simulink library "lib_dGrid"  (R2023b)
settings: Solver=VariableStepAuto  StartTime=0.0  StopTime=10.0  RelTol=1e-3
values from neighbouring files (symbols this model uses):
  C_PM = 10e-3    (= 0.01)    [my_MMC_param.m]
  Cbase = 1/Zbase/wb    (= 3.10849498226e-05)    [my_MMC_param.m]
  f0 = 50/fb    (= 1)    [my_MMC_param.m]
  Fn_filter = 1000    [my_MMC_param.m]
  Fnom = 50    [my_MMC_param.m]
  GFL_APC = 1    [Analysis_Main.m]    (also in initSimu.m; my_MMC_param.m)
  GFL_DVC = 2    [Analysis_Main.m]    (also in initSimu.m; my_MMC_param.m)
  GFM_APC = 3; (values programmed in EMT models)    [Analysis_Main.m]    (also in initSimu.m; my_MMC_param.m = 3)
  GFM_VF = 0    [my_MMC_param.m]
  Ibase = 2*Sbase/(3*Ubase)    [my_MMC_param.m]
  Idcb = Sbase/Udcb    [my_MMC_param.m]
  Ki_Iccsc = 5.15    [my_MMC_param.m]
  Ki_Ireg = CCCTRL.CC.ki    [my_MMC_param.m]
  Ki_Izscc = 100    [my_MMC_param.m]
  Ki_PLL = 1/(CCCTRL.PLL.v0*CCCTRL.PLL.T^2)    [my_MMC_param.m]
  Ki_Preg = 1.0*10    (= 10)    [my_MMC_param.m]
  Ki_Qreg = 1.0*10    (= 10)    [my_MMC_param.m]
  Ki_VAC_GFL = 50    [my_MMC_param.m]
  Ki_VACreg = 10    [my_MMC_param.m]
  Ki_VDCreg = 10    [my_MMC_param.m]
  Ki_WtReg = Kp_WtReg / 0.025    (= 1600)    [my_MMC_param.m]
  Kp_Iccsc = 0.21    [my_MMC_param.m]
  Kp_Ireg = CCCTRL.CC.kp    [my_MMC_param.m]
  Kp_Izscc = 10    [my_MMC_param.m]
  Kp_PLL = 2/CCCTRL.PLL.v0/CCCTRL.PLL.T    [my_MMC_param.m]
  Kp_Preg = 0.5/3*1    (= 0.166666666667)    [my_MMC_param.m]
  Kp_Qreg = 0.5/3*1    (= 0.166666666667)    [my_MMC_param.m]
  Kp_VAC_GFL = 0.5    [my_MMC_param.m]
  Kp_VACreg = 0.01    [my_MMC_param.m]
  Kp_VDCreg = 1    [my_MMC_param.m]
  Kp_WtReg = 40    [my_MMC_param.m]
  Kpv_GFM = 1    [my_MMC_param.m]
  Kpwm = 0.5    [my_MMC_param.m]
  Larm = Larm_pu*(Zbase/wb)    (= 0.0488923985178)    [my_MMC_param.m]
  Lff = Larm_pu/2    (= 0.075)    [my_MMC_param.m]
  Limits_Ireg = [ 2.0  -2.0]    [my_MMC_param.m]
  Limits_Preg = [ 2, -2 ]    [my_MMC_param.m]
  Limits_Qreg = 2*[ 0.42, -0.42 ]    [my_MMC_param.m]
  Limits_VACreg = [ 1.3  -1.3]    [my_MMC_param.m]
  Limits_VDCreg = [ 2.0  -2.0]    [my_MMC_param.m]
  MMC1 = MMC    [Analysis_Main.m]    (also in initSimu.m)
  Nb_PM = 400    [my_MMC_param.m]
  PhaseDelay = 1.0*Ts_Control*2*pi*50    (= 0.0628318530718)    [my_MMC_param.m]
  Pnom = 1000e6    (= 1000000000)    [my_MMC_param.m]
  Rarm = Rarm_pu*Zbase    (= 0.1536)    [my_MMC_param.m]
  Slope_Pref = 0.5    [my_MMC_param.m]
  Slope_Qref = 0.5    [my_MMC_param.m]
  Slope_Vdc_ref = Vnom_dc/2    (= 320000)    [my_MMC_param.m]
  Tdeblock = 1.5    [my_MMC_param.m]
  Ton_CROSSreg = Ton_PQreg+3    (= 7)    [my_MMC_param.m]
  Ton_PQreg = 4    [my_MMC_param.m]
  Ton_VDCreg = 1.5    [my_MMC_param.m]
  Ts = Ts_Control    (= 0.0002)    [my_MMC_param.m]
  Ts_Control = Ts_Power*2    (= 0.0002)    [my_MMC_param.m]
  Ts_Power = 20e-6 * 5    (= 0.0001)    [my_MMC_param.m]
  Ubase = sqrt(2/3)*Vnom_sec    [my_MMC_param.m]
  Udcb = 2*Ubase    [my_MMC_param.m]
  Vc0_PM = 0    [my_MMC_param.m]
  Vnom_dc = 640e3    (= 640000)    [my_MMC_param.m]
  Vnom_sec = 320e3    (= 320000)    [my_MMC_param.m]
  wb = 2*pi*fb    (= 314.159265359)    [my_MMC_param.m]
  Wt_ref_pu = 0.5 * C_PM * (Vnom_dc/Nb_PM)^2 * Nb_PM * 6 / Pnom    (= 0.03072)    [my_MMC_param.m]
undefined symbols (not defined in the file or in its folder): ControlSampleTime, DiscIntNeverNeededParam, MMC, PLL, VSM
libraries: simulink x50, spsCurrentMeasurementLib x20, spsSecondOrderFilterLib x20, spsDiodeLib x12, spsControlledVoltageSourceLib x12, spsSeriesRLCBranchLib x10, spsFirstOrderFilterLib x9, spsVoltageMeasurementLib x8, spsMeanLib x7, FriedrichLibrary x6, $bdroot x6, powerlib_extras x4
(part 8 of 8)

== system lib_dGrid/MMC-configurable control modes/MMC Control/PLL, Measurements and Transformation/from DDSRF-PLL/PT1 as IIR1 ==
  U : Inport
  Gain : Gain  Gain=K*T/(T+2*tau)  SampleTime=T
  Gain1 : Gain  Gain=K*T/(T+2*tau)
  Gain2 : Gain  Gain=(T-2*tau)/(T+2*tau)
  Sum : Sum  Inputs=|++
  Sum1 : Sum  Inputs=+|-
  Unit Delay : UnitDelay  InitialCondition=Init  SampleTime=T  HasFrameUpgradeWarning=on
  Unit Delay1 : UnitDelay  InitialCondition=Init*K  SampleTime=T  HasFrameUpgradeWarning=on
  Y : Outport  VectorParamsAs1DForOutWhenUnconnected=off
  wires:
  Gain2/1 -> Sum1/2
  Sum1/1 -> Sum/2
  Gain1/1 -> Sum1/1
  Unit Delay1/1 -> Gain2/1
  Sum/1 -> Y/1, Unit Delay1/1
  Gain/1 -> Sum/1
  Unit Delay/1 -> Gain1/1
  U/1 -> Gain/1, Unit Delay/1

== system lib_dGrid/MMC-configurable control modes/MMC Control/PLL, Measurements and Transformation/from DDSRF-PLL/ab0->dq0 SinCos ==
  ab0 : Inport
  sincos : Inport  Port=2
  Demux : Demux  Outputs=3
  Demux1 : Demux  Outputs=2
  Mux : Mux  Inputs=3
  Product{,1..3} (4 alike) : Product
  Subtract : Sum
  Subtract1 : Sum  Inputs=-+
  dq0 : Outport  VectorParamsAs1DForOutWhenUnconnected=off
  wires:
  Mux/1 -> dq0/1
  Demux/3 -> Mux/3
  Demux/1 -> Product2/2, Product/2
  ab0/1 -> Demux/1
  sincos/1 -> Demux1/1
  Demux/2 -> Product1/2, Product3/2
  Demux1/2 -> Product3/1, Product/1
  Demux1/1 -> Product2/1, Product1/1
  Product/1 -> Subtract/1
  Product1/1 -> Subtract/2
  Product2/1 -> Subtract1/1
  Product3/1 -> Subtract1/2
  Subtract1/1 -> Mux/2
  Subtract/1 -> Mux/1

== system lib_dGrid/MMC-configurable control modes/MMC Control/PLL, Measurements and Transformation/from DDSRF-PLL/ab0->dq0 SinCos  ==
  ab0 : Inport
  sincos : Inport  Port=2
  Demux : Demux  Outputs=3
  Demux1 : Demux  Outputs=2
  Mux : Mux  Inputs=3
  Product{,1..3} (4 alike) : Product
  Subtract : Sum
  Subtract1 : Sum  Inputs=-+
  dq0 : Outport  VectorParamsAs1DForOutWhenUnconnected=off
  wires:
  Mux/1 -> dq0/1
  Demux/3 -> Mux/3
  Demux/1 -> Product2/2, Product/2
  ab0/1 -> Demux/1
  sincos/1 -> Demux1/1
  Demux/2 -> Product1/2, Product3/2
  Demux1/2 -> Product3/1, Product/1
  Demux1/1 -> Product2/1, Product1/1
  Product/1 -> Subtract/1
  Product1/1 -> Subtract/2
  Product2/1 -> Subtract1/1
  Product3/1 -> Subtract1/2
  Subtract1/1 -> Mux/2
  Subtract/1 -> Mux/1

== system lib_dGrid/MMC-configurable control modes/MMC Control/PLL, Measurements and Transformation/from DDSRF-PLL/dq0->ab0 SinCos ==
  ab0 : Inport
  sincos : Inport  Port=2
  Demux : Demux  Outputs=3
  Demux1 : Demux  Outputs=2
  Mux : Mux  Inputs=3
  Product{,1..3} (4 alike) : Product
  Subtract : Sum  Inputs=+-
  Subtract1 : Sum
  dq0 : Outport  VectorParamsAs1DForOutWhenUnconnected=off
  wires:
  Subtract/1 -> Mux/1
  Subtract1/1 -> Mux/2
  Product3/1 -> Subtract1/2
  Product2/1 -> Subtract1/1
  Product1/1 -> Subtract/2
  Product/1 -> Subtract/1
  Demux1/1 -> Product1/1, Product2/1
  Demux1/2 -> Product/1, Product3/1
  Demux/2 -> Product3/2, Product1/2
  sincos/1 -> Demux1/1
  ab0/1 -> Demux/1
  Demux/1 -> Product/2, Product2/2
  Demux/3 -> Mux/3
  Mux/1 -> dq0/1

== system lib_dGrid/MMC-configurable control modes/MMC Control/PLL, Measurements and Transformation/from DDSRF-PLL/dq0->ab0 SinCos  ==
  ab0 : Inport
  sincos : Inport  Port=2
  Demux : Demux  Outputs=3
  Demux1 : Demux  Outputs=2
  Mux : Mux  Inputs=3
  Product{,1..3} (4 alike) : Product
  Subtract : Sum  Inputs=+-
  Subtract1 : Sum
  dq0 : Outport  VectorParamsAs1DForOutWhenUnconnected=off
  wires:
  Subtract/1 -> Mux/1
  Subtract1/1 -> Mux/2
  Product3/1 -> Subtract1/2
  Product2/1 -> Subtract1/1
  Product1/1 -> Subtract/2
  Product/1 -> Subtract/1
  Demux1/1 -> Product1/1, Product2/1
  Demux1/2 -> Product/1, Product3/1
  Demux/2 -> Product3/2, Product1/2
  sincos/1 -> Demux1/1
  ab0/1 -> Demux/1
  Demux/1 -> Product/2, Product2/2
  Demux/3 -> Mux/3
  Mux/1 -> dq0/1

== system lib_dGrid/MMC-configurable control modes/MMC Control/VSM Control/Inner Loop Control/CC ==
  Error : Inport  SampleTime=Ts
  Discrete-Time Integrator : DiscreteIntegrator  InitialCondition=Init  SampleTime=Ts  LimitOutput=on  UpperSaturationLimit=UpperLimit  LowerSaturationLimit=LowerLimit  ICPrevOutput=DiscIntNeverNeededParam  ICPrevScaledInput=DiscIntNeverNeededParam
  Kp4 : Gain  Gain=Kp  SaturateOnIntegerOverflow=on  SampleTime=Ts  OutDataTypeStr=Inherit: Same as input  ParamDataTypeStr=Inherit: Same as input
  Kp5 : Gain  Gain=Ki  SaturateOnIntegerOverflow=on  SampleTime=Ts  OutDataTypeStr=Inherit: Same as input  ParamDataTypeStr=Inherit: Same as input
  Saturation2 : Saturate  UpperLimit=UpperLimit  LowerLimit=LowerLimit  SampleTime=Ts
  Sum6 : Sum  InputSameDT=on  SaturateOnIntegerOverflow=on  SampleTime=Ts  OutDataTypeStr=Inherit: Same as first input
  Zero-Order Hold : ZeroOrderHold  SampleTime=Ts
  Out : Outport  SampleTime=Ts  InitialOutput=0  VectorParamsAs1DForOutWhenUnconnected=off
  wires:
  Zero-Order Hold/1 -> Sum6/1
  Error/1 -> Kp5/1, Kp4/1
  Sum6/1 -> Saturation2/1
  Kp4/1 -> Zero-Order Hold/1
  Discrete-Time Integrator/1 -> Sum6/2
  Saturation2/1 -> Out/1
  Kp5/1 -> Discrete-Time Integrator/1

== system lib_dGrid/MMC-configurable control modes/MMC Control/VSM Control/Inner Loop Control/CC  ==
  Error : Inport  SampleTime=Ts
  Discrete-Time Integrator : DiscreteIntegrator  InitialCondition=Init  SampleTime=Ts  LimitOutput=on  UpperSaturationLimit=UpperLimit  LowerSaturationLimit=LowerLimit  ICPrevOutput=DiscIntNeverNeededParam  ICPrevScaledInput=DiscIntNeverNeededParam
  Kp4 : Gain  Gain=Kp  SaturateOnIntegerOverflow=on  SampleTime=Ts  OutDataTypeStr=Inherit: Same as input  ParamDataTypeStr=Inherit: Same as input
  Kp5 : Gain  Gain=Ki  SaturateOnIntegerOverflow=on  SampleTime=Ts  OutDataTypeStr=Inherit: Same as input  ParamDataTypeStr=Inherit: Same as input
  Saturation2 : Saturate  UpperLimit=UpperLimit  LowerLimit=LowerLimit  SampleTime=Ts
  Sum6 : Sum  InputSameDT=on  SaturateOnIntegerOverflow=on  SampleTime=Ts  OutDataTypeStr=Inherit: Same as first input
  Zero-Order Hold : ZeroOrderHold  SampleTime=Ts
  Out : Outport  SampleTime=Ts  InitialOutput=0  VectorParamsAs1DForOutWhenUnconnected=off
  wires:
  Zero-Order Hold/1 -> Sum6/1
  Error/1 -> Kp5/1, Kp4/1
  Sum6/1 -> Saturation2/1
  Kp4/1 -> Zero-Order Hold/1
  Discrete-Time Integrator/1 -> Sum6/2
  Saturation2/1 -> Out/1
  Kp5/1 -> Discrete-Time Integrator/1

== system lib_dGrid/MMC-configurable control modes/MMC Control/VSM Control/VSM1/Angle Integrator [SI] ==
  omega : Inport
  phi0 : Inport  Port=2
  Bias : Bias  Bias=-2*pi  SaturateOnIntegerOverflow=off
  Bias1 : Bias  Bias=2*pi  SaturateOnIntegerOverflow=off
  Delay : Delay  DelayLength=1  InitialConditionSource=Input port  SampleTime=Ts
      settings: InputPortMap=u0,p4
  Gain3 : Gain  Gain=Ts
  Sum : Sum  Inputs=|++
  Switch : Switch  Criteria=u2 > Threshold  Threshold=pi  SaturateOnIntegerOverflow=off  InputSameDT=off
  Switch1 : Switch  Threshold=-pi  SaturateOnIntegerOverflow=off  InputSameDT=off
  phi : Outport  VectorParamsAs1DForOutWhenUnconnected=off
  wires:
  Switch1/1 -> Delay/1
  Bias1/1 -> Switch1/3
  Switch/1 -> Switch1/2, Bias1/1, Switch1/1
  Delay/1 -> phi/1, Sum/2
  Sum/1 -> Bias/1, Switch/2, Switch/3
  Bias/1 -> Switch/1
  Gain3/1 -> Sum/1
  omega/1 -> Gain3/1
  phi0/1 -> Delay/2

== system lib_dGrid/MMC-configurable control modes/MMC Control/VSM Control/Virtual circuit daniel style1/transient rv (HP)1 -dd's form ==
  In1 : Inport
  Add : Sum  Inputs=+-
  Constant : Constant  Value=tau
  Delay2 : Delay  DelayLength=1  SampleTime=TS
  Divide : Product  Inputs=*/
  Gain : Gain  Gain=TS
  Gain1 : Gain
  Sum : Sum  Inputs=|++
  Sum2 : Sum  Inputs=|+-
  Out1 : Outport  VectorParamsAs1DForOutWhenUnconnected=off
  wires:
  Delay2/1 -> Add/2, Sum/2, Sum2/2
  Gain1/1 -> Add/1
  Sum/1 -> Delay2/1
  In1/1 -> Sum2/1, Gain1/1
  Add/1 -> Out1/1
  Divide/1 -> Sum/1
  Constant/1 -> Divide/2
  Sum2/1 -> Gain/1
  Gain/1 -> Divide/1

== system lib_dGrid/MMC-configurable control modes/MMC Control/VSM Control/Virtual circuit daniel style1/transient rv (HP)1 yz's form ==
  In1 : Inport
  Add : Sum  Inputs=+-
  Gain1 : Gain
  Low-Pass Filter (Discrete or Continuous) : eeGeneralControl/Low-Pass Filter (Discrete or Continuous)  K=1  T=tau  B=inf  A=-inf  init_option=Inherited from block input  x0=0  Ts=TS
  Out1 : Outport  VectorParamsAs1DForOutWhenUnconnected=off
  wires:
  Gain1/1 -> Add/1
  In1/1 -> Low-Pass Filter (Discrete or Continuous)/1, Gain1/1
  Add/1 -> Out1/1
  Low-Pass Filter (Discrete or Continuous)/1 -> Add/2

== system lib_dGrid/MMC-configurable control modes/MMC Control/VSM Control/Virtual circuit daniel style1/transient rv (HP)2 (dd's form) ==
  In1 : Inport
  Add : Sum  Inputs=+-
  Constant : Constant  Value=tau
  Delay2 : Delay  DelayLength=1  SampleTime=TS
  Divide : Product  Inputs=*/
  Gain : Gain  Gain=TS
  Gain1 : Gain
  Sum : Sum  Inputs=|++
  Sum2 : Sum  Inputs=|+-
  Out1 : Outport  VectorParamsAs1DForOutWhenUnconnected=off
  wires:
  Gain/1 -> Divide/1
  Sum2/1 -> Gain/1
  Constant/1 -> Divide/2
  Divide/1 -> Sum/1
  Add/1 -> Out1/1
  In1/1 -> Gain1/1, Sum2/1
  Sum/1 -> Delay2/1
  Gain1/1 -> Add/1
  Delay2/1 -> Sum2/2, Sum/2, Add/2

== system lib_dGrid/TL-VSC-configurable control modes/VSC Control/PLL, Measurements and Transformation/Symmetrical PLL/Angle Integrator [SI] ==
  omega : Inport
  phi0 : Inport  Port=2
  Bias : Bias  Bias=-2*pi  SaturateOnIntegerOverflow=off
  Bias1 : Bias  Bias=2*pi  SaturateOnIntegerOverflow=off
  Delay : Delay  DelayLength=1  InitialConditionSource=Input port  SampleTime=Ts
      settings: InputPortMap=u0,p4
  Gain3 : Gain  Gain=Ts
  Sum : Sum  Inputs=|++
  Switch : Switch  Criteria=u2 > Threshold  Threshold=pi  SaturateOnIntegerOverflow=off  InputSameDT=off
  Switch1 : Switch  Threshold=-pi  SaturateOnIntegerOverflow=off  InputSameDT=off
  phi : Outport  VectorParamsAs1DForOutWhenUnconnected=off
  wires:
  Switch1/1 -> Delay/1
  Bias1/1 -> Switch1/3
  Switch/1 -> Switch1/2, Bias1/1, Switch1/1
  Delay/1 -> phi/1, Sum/2
  Sum/1 -> Bias/1, Switch/2, Switch/3
  Bias/1 -> Switch/1
  Gain3/1 -> Sum/1
  omega/1 -> Gain3/1
  phi0/1 -> Delay/2

== system lib_dGrid/TL-VSC-configurable control modes/VSC Control/PLL, Measurements and Transformation/Symmetrical PLL/PhN->ab0 ==
  PhN : Inport
  AlphaBetaNull Transformation : Gain  Gain="[2/3   -1/3    -1/3;   0   1/sqrt(3) -1/sqrt(3); 1/3 1/3 1/3]"  Multiplication=Matrix(K*u) (u vector)
  ab0 : Outport  VectorParamsAs1DForOutWhenUnconnected=off
  wires:
  AlphaBetaNull Transformation/1 -> ab0/1
  PhN/1 -> AlphaBetaNull Transformation/1

== system lib_dGrid/TL-VSC-configurable control modes/VSC Control/PLL, Measurements and Transformation/Symmetrical PLL/ab0->dq0-faster ==
  ab0 : Inport
  w : Inport  Port=2
  Demux : Demux  Outputs=3
  Mux : Mux  Inputs=3
  Product{,1..3} (4 alike) : Product
  Subtract : Sum
  Subtract1 : Sum  Inputs=-+
  Trigonometric Function : Trigonometry  Operator=sincos
  dq0 : Outport  VectorParamsAs1DForOutWhenUnconnected=off
  wires:
  Subtract/1 -> Mux/1
  Subtract1/1 -> Mux/2
  Product3/1 -> Subtract1/2
  Product2/1 -> Subtract1/1
  Product1/1 -> Subtract/2
  Product/1 -> Subtract/1
  Trigonometric Function/1 -> Product1/1, Product2/1
  Trigonometric Function/2 -> Product3/1, Product/1
  Demux/2 -> Product3/2, Product1/2
  w/1 -> Trigonometric Function/1
  ab0/1 -> Demux/1
  Demux/1 -> Product/2, Product2/2
  Demux/3 -> Mux/3
  Mux/1 -> dq0/1

== system lib_dGrid/TL-VSC-configurable control modes/VSC Control/PLL, Measurements and Transformation/Symmetrical PLL/discrete PID ==
  e : Inport
  Gain : Gain  Gain=Kp
  Gain1 : Gain  Gain=Ki*Ts
  Gain2 : Gain  Gain=Kd/Ts
  Sum1 : Sum  Inputs=+++
  Sum2 : Sum  Inputs=|++
  Sum3 : Sum  Inputs=|-+
  Unit Delay2 : UnitDelay  SampleTime=Ts  HasFrameUpgradeWarning=on
  Unit Delay3 : UnitDelay  InitialCondition=x_init  SampleTime=Ts  HasFrameUpgradeWarning=on
  y : Outport  VectorParamsAs1DForOutWhenUnconnected=off
  wires:
  e/1 -> Gain/1, Gain1/1, Unit Delay2/1, Sum3/1
  Unit Delay2/1 -> Sum3/2
  Sum1/1 -> y/1
  Gain/1 -> Sum1/1
  Unit Delay3/1 -> Sum1/2, Sum2/2
  Gain2/1 -> Sum1/3
  Gain1/1 -> Sum2/1
  Sum3/1 -> Gain2/1
  Sum2/1 -> Unit Delay3/1

== system lib_dGrid/TL-VSC-configurable control modes/VSC Control/VSM Control/Inner Loop Control/CC ==
  Error : Inport  SampleTime=Ts
  Discrete-Time Integrator : DiscreteIntegrator  InitialCondition=Init  SampleTime=Ts  LimitOutput=on  UpperSaturationLimit=UpperLimit  LowerSaturationLimit=LowerLimit  ICPrevOutput=DiscIntNeverNeededParam  ICPrevScaledInput=DiscIntNeverNeededParam
  Kp4 : Gain  Gain=Kp  SaturateOnIntegerOverflow=on  SampleTime=Ts  OutDataTypeStr=Inherit: Same as input  ParamDataTypeStr=Inherit: Same as input
  Kp5 : Gain  Gain=Ki  SaturateOnIntegerOverflow=on  SampleTime=Ts  OutDataTypeStr=Inherit: Same as input  ParamDataTypeStr=Inherit: Same as input
  Saturation2 : Saturate  UpperLimit=UpperLimit  LowerLimit=LowerLimit  SampleTime=Ts
  Sum6 : Sum  InputSameDT=on  SaturateOnIntegerOverflow=on  SampleTime=Ts  OutDataTypeStr=Inherit: Same as first input
  Zero-Order Hold : ZeroOrderHold  SampleTime=Ts
  Out : Outport  SampleTime=Ts  InitialOutput=0  VectorParamsAs1DForOutWhenUnconnected=off
  wires:
  Zero-Order Hold/1 -> Sum6/1
  Error/1 -> Kp5/1, Kp4/1
  Sum6/1 -> Saturation2/1
  Kp4/1 -> Zero-Order Hold/1
  Discrete-Time Integrator/1 -> Sum6/2
  Saturation2/1 -> Out/1
  Kp5/1 -> Discrete-Time Integrator/1

== system lib_dGrid/TL-VSC-configurable control modes/VSC Control/VSM Control/Inner Loop Control/CC  ==
  Error : Inport  SampleTime=Ts
  Discrete-Time Integrator : DiscreteIntegrator  InitialCondition=Init  SampleTime=Ts  LimitOutput=on  UpperSaturationLimit=UpperLimit  LowerSaturationLimit=LowerLimit  ICPrevOutput=DiscIntNeverNeededParam  ICPrevScaledInput=DiscIntNeverNeededParam
  Kp4 : Gain  Gain=Kp  SaturateOnIntegerOverflow=on  SampleTime=Ts  OutDataTypeStr=Inherit: Same as input  ParamDataTypeStr=Inherit: Same as input
  Kp5 : Gain  Gain=Ki  SaturateOnIntegerOverflow=on  SampleTime=Ts  OutDataTypeStr=Inherit: Same as input  ParamDataTypeStr=Inherit: Same as input
  Saturation2 : Saturate  UpperLimit=UpperLimit  LowerLimit=LowerLimit  SampleTime=Ts
  Sum6 : Sum  InputSameDT=on  SaturateOnIntegerOverflow=on  SampleTime=Ts  OutDataTypeStr=Inherit: Same as first input
  Zero-Order Hold : ZeroOrderHold  SampleTime=Ts
  Out : Outport  SampleTime=Ts  InitialOutput=0  VectorParamsAs1DForOutWhenUnconnected=off
  wires:
  Zero-Order Hold/1 -> Sum6/1
  Error/1 -> Kp5/1, Kp4/1
  Sum6/1 -> Saturation2/1
  Kp4/1 -> Zero-Order Hold/1
  Discrete-Time Integrator/1 -> Sum6/2
  Saturation2/1 -> Out/1
  Kp5/1 -> Discrete-Time Integrator/1

== system lib_dGrid/TL-VSC-configurable control modes/VSC Control/VSM Control/VSM1/Angle Integrator [SI] ==
  omega : Inport
  phi0 : Inport  Port=2
  Bias : Bias  Bias=-2*pi  SaturateOnIntegerOverflow=off
  Bias1 : Bias  Bias=2*pi  SaturateOnIntegerOverflow=off
  Delay : Delay  DelayLength=1  InitialConditionSource=Input port  SampleTime=Ts
      settings: InputPortMap=u0,p4
  Gain3 : Gain  Gain=Ts
  Sum : Sum  Inputs=|++
  Switch : Switch  Criteria=u2 > Threshold  Threshold=pi  SaturateOnIntegerOverflow=off  InputSameDT=off
  Switch1 : Switch  Threshold=-pi  SaturateOnIntegerOverflow=off  InputSameDT=off
  phi : Outport  VectorParamsAs1DForOutWhenUnconnected=off
  wires:
  Switch1/1 -> Delay/1
  Bias1/1 -> Switch1/3
  Switch/1 -> Switch1/2, Bias1/1, Switch1/1
  Delay/1 -> phi/1, Sum/2
  Sum/1 -> Bias/1, Switch/2, Switch/3
  Bias/1 -> Switch/1
  Gain3/1 -> Sum/1
  omega/1 -> Gain3/1
  phi0/1 -> Delay/2

== system lib_dGrid/TL-VSC-configurable control modes/VSC Control/VSM Control/Virtual circuit daniel style1/transient rv (HP)1 -dd's form ==
  In1 : Inport
  Add : Sum  Inputs=+-
  Constant : Constant  Value=tau
  Delay2 : Delay  DelayLength=1  SampleTime=TS
  Divide : Product  Inputs=*/
  Gain : Gain  Gain=TS
  Gain1 : Gain
  Sum : Sum  Inputs=|++
  Sum2 : Sum  Inputs=|+-
  Out1 : Outport  VectorParamsAs1DForOutWhenUnconnected=off
  wires:
  Delay2/1 -> Add/2, Sum/2, Sum2/2
  Gain1/1 -> Add/1
  Sum/1 -> Delay2/1
  In1/1 -> Sum2/1, Gain1/1
  Add/1 -> Out1/1
  Divide/1 -> Sum/1
  Constant/1 -> Divide/2
  Sum2/1 -> Gain/1
  Gain/1 -> Divide/1

== system lib_dGrid/TL-VSC-configurable control modes/VSC Control/VSM Control/Virtual circuit daniel style1/transient rv (HP)1 yz's form ==
  In1 : Inport
  Add : Sum  Inputs=+-
  Gain1 : Gain
  Low-Pass Filter (Discrete or Continuous) : eeGeneralControl/Low-Pass Filter (Discrete or Continuous)  K=1  T=tau  B=inf  A=-inf  init_option=Inherited from block input  x0=0  Ts=TS
  Out1 : Outport  VectorParamsAs1DForOutWhenUnconnected=off
  wires:
  Gain1/1 -> Add/1
  In1/1 -> Low-Pass Filter (Discrete or Continuous)/1, Gain1/1
  Add/1 -> Out1/1
  Low-Pass Filter (Discrete or Continuous)/1 -> Add/2

== system lib_dGrid/TL-VSC-configurable control modes/VSC Control/VSM Control/Virtual circuit daniel style1/transient rv (HP)2 (dd's form) ==
  In1 : Inport
  Add : Sum  Inputs=+-
  Constant : Constant  Value=tau
  Delay2 : Delay  DelayLength=1  SampleTime=TS
  Divide : Product  Inputs=*/
  Gain : Gain  Gain=TS
  Gain1 : Gain
  Sum : Sum  Inputs=|++
  Sum2 : Sum  Inputs=|+-
  Out1 : Outport  VectorParamsAs1DForOutWhenUnconnected=off
  wires:
  Gain/1 -> Divide/1
  Sum2/1 -> Gain/1
  Constant/1 -> Divide/2
  Divide/1 -> Sum/1
  Add/1 -> Out1/1
  In1/1 -> Gain1/1, Sum2/1
  Sum/1 -> Delay2/1
  Gain1/1 -> Add/1
  Delay2/1 -> Sum2/2, Sum/2, Add/2

== system lib_dGrid/MMC-configurable control modes/MMC Control/CCSC + ZSCC control/Subsystem/EnergyCalc/PhN->ab2 ==
  PhN : Inport
  AlphaBetaNull Transformation : Gain  Gain="[2/3   -1/3    -1/3;   0   1/sqrt(3) -1/sqrt(3); 1/3 1/3 1/3]"  Multiplication=Matrix(K*u) (u vector)
  ab0 : Outport  VectorParamsAs1DForOutWhenUnconnected=off
  wires:
  AlphaBetaNull Transformation/1 -> ab0/1
  PhN/1 -> AlphaBetaNull Transformation/1

== system lib_dGrid/MMC-configurable control modes/MMC Control/CCSC + ZSCC control/Subsystem/EnergyCalc/ab0->dq0-faster1 ==
  ab0 : Inport
  w : Inport  Port=2
  Demux : Demux  Outputs=3
  Mux : Mux  Inputs=3
  Product{,1..3} (4 alike) : Product
  Subtract : Sum
  Subtract1 : Sum  Inputs=-+
  Trigonometric Function : Trigonometry  Operator=sincos
  dq0 : Outport  VectorParamsAs1DForOutWhenUnconnected=off
  wires:
  Subtract/1 -> Mux/1
  Subtract1/1 -> Mux/2
  Product3/1 -> Subtract1/2
  Product2/1 -> Subtract1/1
  Product1/1 -> Subtract/2
  Product/1 -> Subtract/1
  Trigonometric Function/1 -> Product1/1, Product2/1
  Trigonometric Function/2 -> Product3/1, Product/1
  Demux/2 -> Product3/2, Product1/2
  w/1 -> Trigonometric Function/1
  ab0/1 -> Demux/1
  Demux/1 -> Product/2, Product2/2
  Demux/3 -> Mux/3
  Mux/1 -> dq0/1
